simulink model "Heat_Test"  (R2018b)
settings: Solver=VariableStepAuto  StartTime=0.0  StopTime=100  RelTol=1e-3
values from neighbouring files (symbols this model uses):
  air_data = load('air_data.csv')    [eqns_motion_script.m]    (also in eqns_motion_script_439.m)
libraries: aerolibatmos2 x1
settings Model: Creator=bartk  LastModifiedBy=bartk

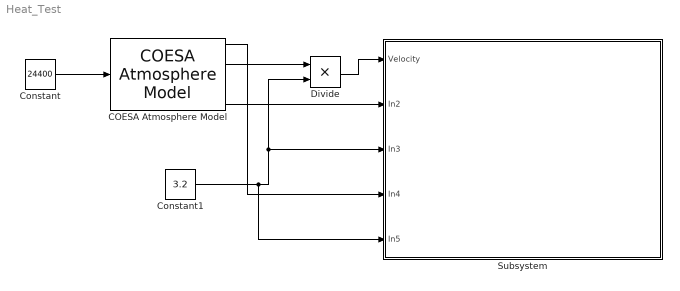
== system Heat_Test ==
  COESA Atmosphere Model : aerolibatmos2/COESA Atmosphere Model  units=Metric (MKS)  spec=1976 COESA-extended U.S. Standard Atmosphere  model=Profile  profile_var=High temperature  profile_percent=1%  profile_alt=5 km (16404 ft)  envelope_var=High temperature  envelope_percent=1%  action=Warning
  Constant : Constant  Value=24400
  Constant1 : Constant  Value=3.2
  Divide : Product  Inputs=**
  Subsystem : Subsystem
  wires:
  Constant/1 -> COESA Atmosphere Model/1
  COESA Atmosphere Model/2 -> Divide/1
  Constant1/1 -> Subsystem/5(In5), Divide/2, Subsystem/3(In3)
  Divide/1 -> Subsystem/1(Velocity)
  COESA Atmosphere Model/4 -> Subsystem/2(In2)
  COESA Atmosphere Model/1 -> Subsystem/4(In4)

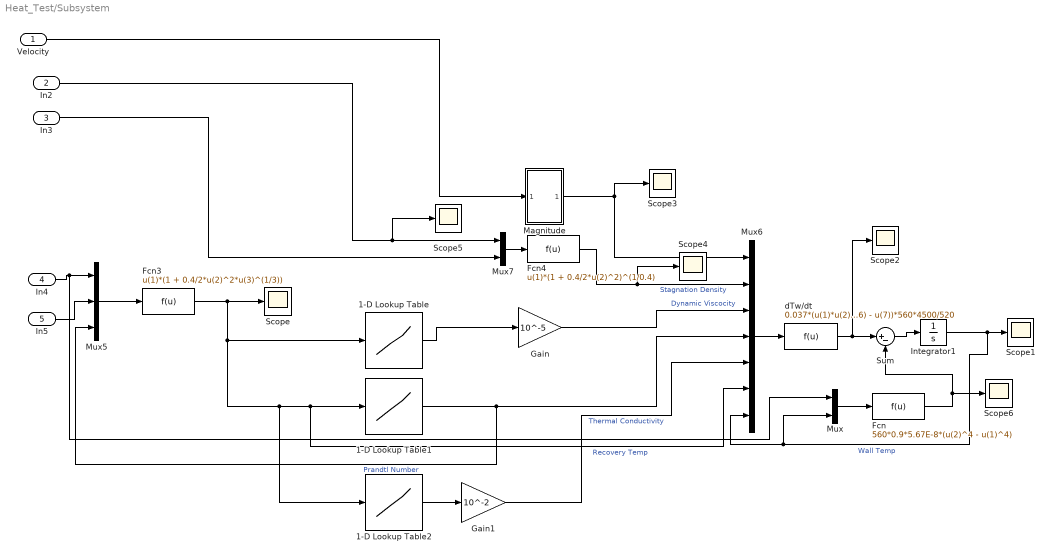
== system Heat_Test/Subsystem ==
  Velocity : Inport
  In2 : Inport  Port=2
  In3 : Inport  Port=3
  In4 : Inport  Port=4
  In5 : Inport  Port=5
  1-D Lookup Table : Lookup_n-D  NumberOfTableDimensions=1  BreakpointsForDimension1=air_data(:,1)  Table=air_data(:,5)  InternalRulePriority=Speed  RndMeth=Simplest  InputSameDT=on
  1-D Lookup Table1 : Lookup_n-D  NumberOfTableDimensions=1  BreakpointsForDimension1=air_data(:,1)  Table=air_data(:,7)  InternalRulePriority=Speed  RndMeth=Simplest  InputSameDT=on
  1-D Lookup Table2 : Lookup_n-D  NumberOfTableDimensions=1  BreakpointsForDimension1=air_data(:,1)  Table=air_data(:,6)  InternalRulePriority=Speed  RndMeth=Simplest  InputSameDT=on
  Fcn : Fcn  Expr=560*0.9*5.67E-8*(u(2)^4 - u(1)^4)
  Fcn3 : Fcn  Expr=u(1)*(1 + 0.4/2*u(2)^2*u(3)^(1/3))
  Fcn4 : Fcn  Expr=u(1)*(1 + 0.4/2*u(2)^2)^(1/0.4)
  Gain : Gain  Gain=10^-5
  Gain1 : Gain  Gain=10^-2
  Integrator1 : Integrator  InitialCondition=300
  Magnitude : Subsystem
  Mux : Mux  Inputs=2
  Mux5 : Mux  Inputs=3
  Mux6 : Mux  Inputs=7
  Mux7 : Mux  Inputs=2
  Scope{,1..6} (7 alike) : Scope
  Sum : Sum  Inputs=|+-
  dTw/dt : Fcn  Expr=0.037*(u(1)*u(2)*32.6/u(3))^(4/5)*u(4)^(1/3)*u(5)*(u(6) - u(7))*560*4500/520
  wires:
  Mux6/1 -> dTw/dt/1
  Gain1/1 -> Mux6/5  "Thermal Conductivity"
  Mux5/1 -> Fcn3/1
  dTw/dt/1 -> Sum/1, Scope2/1
  Fcn3/1 -> 1-D Lookup Table2/1, Mux6/6, 1-D Lookup Table1/1, 1-D Lookup Table/1, Scope/1  "Recovery Temp"
  1-D Lookup Table1/1 -> Mux6/4, Mux5/3  "Prandtl Number"
  Mux7/1 -> Fcn4/1
  In2/1 -> Scope5/1, Mux7/1
  In3/1 -> Mux7/2
  1-D Lookup Table2/1 -> Gain1/1
  Gain/1 -> Mux6/3  "Dynamic Viscocity"
  Integrator1/1 -> Mux/2, Mux6/7, Scope1/1  "Wall Temp"
  Fcn4/1 -> Scope4/1, Mux6/2  "Stagnation Density"
  In5/1 -> Mux5/2
  Magnitude/1(Out1) -> Mux6/1, Scope3/1
  1-D Lookup Table/1 -> Gain/1
  Velocity/1 -> Magnitude/1(Velocity)
  In4/1 -> Mux/1, Mux5/1
  Sum/1 -> Integrator1/1
  Mux/1 -> Fcn/1
  Fcn/1 -> Scope6/1, Sum/2

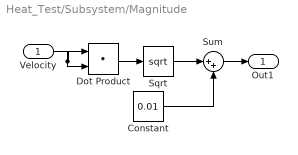
== system Heat_Test/Subsystem/Magnitude ==
  Velocity : Inport
  Constant : Constant  Value=0.01
  Dot Product : DotProduct  InputSameDT=on  OutDataTypeStr=Inherit: Inherit via internal rule
  Sqrt : Sqrt  SaturateOnIntegerOverflow=on
  Sum : Sum  Inputs=|++
  Out1 : Outport
  wires:
  Sum/1 -> Out1/1
  Velocity/1 -> Dot Product/2, Dot Product/1
  Dot Product/1 -> Sqrt/1
  Constant/1 -> Sum/2
  Sqrt/1 -> Sum/1
